simulink library "HexapodLib"  (R2014b)
settings: Solver=ode45  StartTime=0.0  StopTime=10.0  RelTol=1e-3
undefined symbols (not defined in the file): X, Y, Z
libraries: nesl_utility x95, sm_lib x85, HexapodLib x15, Contact_Forces_Lib x12
(part 1 of 3)
settings Model: Creator=Sebastian  LastModifiedBy=Sebastian

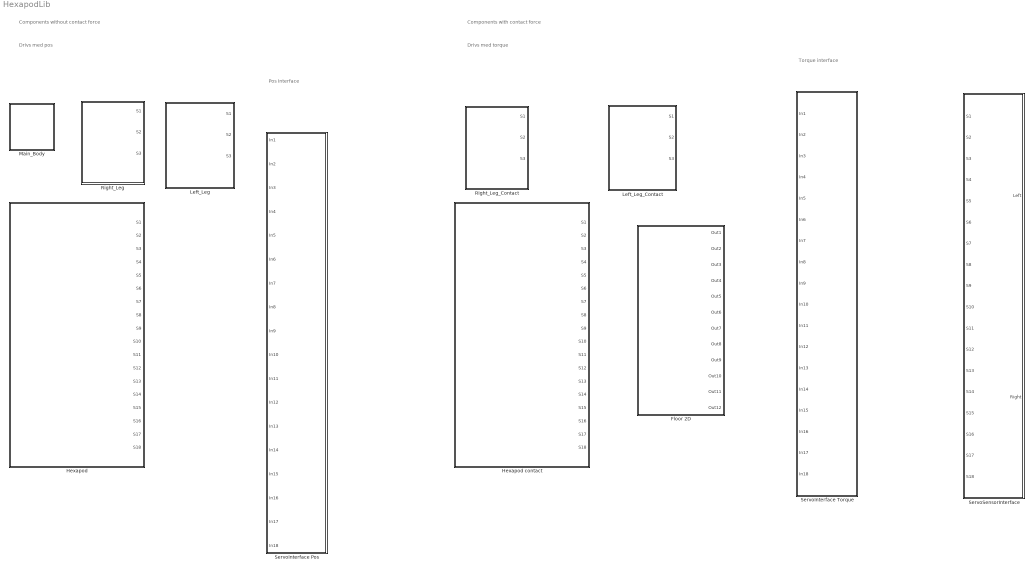
== system HexapodLib ==
  note: Pos Interface
  note: Torque interface
  note: Drivs med pos
  note: Components with contact force
  note: Components without contact force
  note: Drivs med torque
  Floor 2D : Subsystem  mask{my_k=0.5, my_s=0.7, v_th=0.0001}
      mask prompts: my_k "Coefficient of Kinetic Friction"; my_s "Coefficient of Static Friction"; v_th "Velocity Threshold (m/s)"
  Hexapod : Subsystem
  Hexapod contact : Subsystem
  Left_Leg : Subsystem
  Left_Leg_Contact : Subsystem
  Main_Body : Subsystem
  Right_Leg : Subsystem
  Right_Leg_Contact : Subsystem
  ServoInterface Pos : Subsystem  mask{Filter_time=0.001}
      mask prompts: Filter_time "Filter time"
  ServoInterface Torque : Subsystem
  ServoSensorInterface : Subsystem

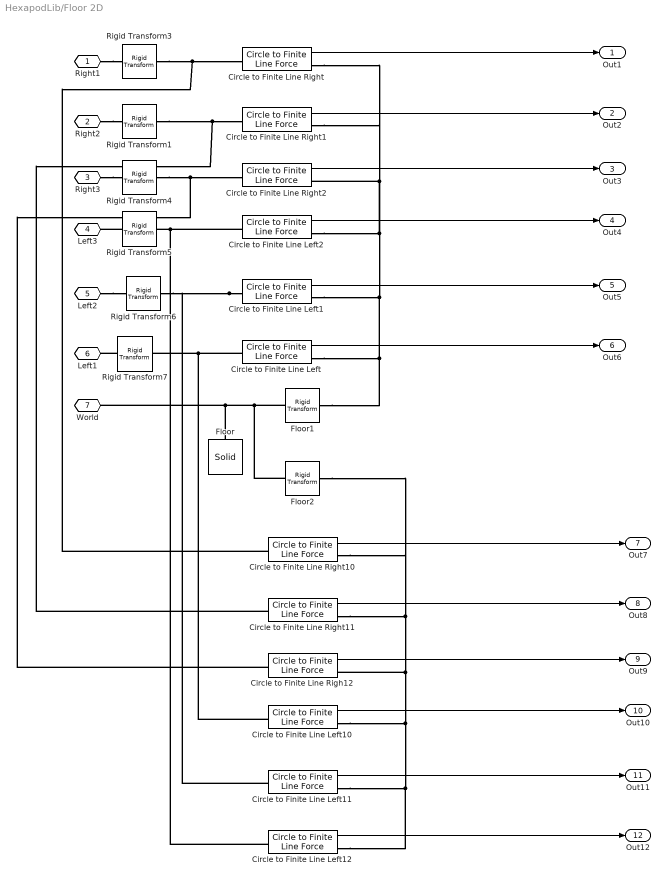
== system HexapodLib/Floor 2D ==
  Circle to Finite Line Left{,1..2,10..12} (6 alike) : Contact_Forces_Lib/2D/Circle to Finite Line Force  circle_rad=0.0048  line_depth=0.05/2  line_length=5  force_law=Linear  k_contact=1e6  b_contact=1e2  pen_full_damp_F=1e-2  pen_exponent=1  custom_param_1=1  custom_param_2=1  friction_law=Stick-Slip Continuous  mu_kinetic=my_k  mu_static=my_s  v_thr=v_th
  Circle to Finite Line Righ12 : Contact_Forces_Lib/2D/Circle to Finite Line Force  circle_rad=0.0048  line_depth=0.05/2  line_length=5  force_law=Linear  k_contact=1e6  b_contact=1e2  pen_full_damp_F=1e-2  pen_exponent=1  custom_param_1=1  custom_param_2=1  friction_law=Stick-Slip Continuous  mu_kinetic=my_k  mu_static=my_s  v_thr=v_th
  Circle to Finite Line Right{,1..2,10..11} (5 alike) : Contact_Forces_Lib/2D/Circle to Finite Line Force  circle_rad=0.0048  line_depth=0.05/2  line_length=5  force_law=Linear  k_contact=1e6  b_contact=1e2  pen_full_damp_F=1e-2  pen_exponent=1  custom_param_1=1  custom_param_2=1  friction_law=Stick-Slip Continuous  mu_kinetic=my_k  mu_static=my_s  v_thr=v_th
  Floor : sm_lib/Body Elements/Solid  InertiaType=CalculateFromGeometry  Mass=1  MassUnits=kg  CenterOfMass=[0 0 0]  CenterOfMassUnits=m  MomentsOfInertia=[1 1 1]  MomentsOfInertiaUnits=kg*m^2  ProductsOfInertia=[0 0 0]  ProductsOfInertiaUnits=kg*m^2  DensityBased=on  Density=1000  DensityUnits=kg/(m^3)  GraphicType=FromGeometry  MarkerShape=Sphere  MarkerSize=10  MarkerSizeUnits=m  GraphicVisPropType=SimpleVisualProperties  GraphicDiffuseColor=[0.4 0.4 0.0]  GraphicSpecularColor=[0.5 0.5 0.5 1.0]  GraphicAmbientColor=[0.15 0.15 0.15 1.0]  GraphicEmissiveColor=[0.0 0.0 0.0 1.0]  GraphicShininess=75  GraphicOpacity=1.0  GeometryShape=Brick  RectangleSize=[1 1]  RectangleSizeUnits=m  BrickDimensions=[3 3 0.05]  BrickDimensionUnits=m  CylinderRadius=1  CylinderRadiusUnits=m  CylinderLength=1  CylinderLengthUnits=m  SphereRadius=1  SphereRadiusUnits=m  EllipsoidRadii=[1 1 1]  EllipsoidRadiiUnits=m  ExtrusionCrossSection=[1 1; -1 1; -1 -1; 1 -1]  ExtrusionCrossSectionUnits=m  ExtrusionLength=1  ExtrusionLengthUnits=m  PolygonNumSides=3  PolygonOuterRadius=1  PolygonOuterRadiusUnits=m  ExtGeomFileType=STL  ExtGeomFileUnits=m  RevolutionCrossSection=[1 1; 1 -1; 2 -1; 2 1]  RevolutionCrossSectionUnits=m  RevolutionExtent=Full  RevolutionAngle=180  RevolutionAngleUnits=deg  BlockFunction=simmechanics.library.body_elements.solid
  Floor1 : sm_lib/Frames and Transforms/Rigid Transform  TranslationMethod=None  TranslationLengthUnit=m  TranslationStandardAxis=+Z  TranslationStandardOffset=0  TranslationCartesianOffset=[0 0 0]  TranslationROffset=0  TranslationROffsetUnits=m  TranslationZOffset=0  TranslationZOffsetUnits=m  TranslationThetaOffset=0  TranslationThetaOffsetUnits=deg  RotationMethod=AlignedAxes  RotationAngleUnits=deg  RotationStandardAxis=+Z  RotationAngle=0  RotationArbitraryAxis=[0 0 1]  FollAlignAxisA=+X  BaseAlignAxisA=+Z  FollAlignAxisB=+Y  BaseAlignAxisB=+X  RotationMatrix=[1 0 0; 0 1 0; 0 0 1]  BlockFunction=simmechanics.library.frames_transforms.rigid_transform
  Floor2 : sm_lib/Frames and Transforms/Rigid Transform  TranslationMethod=None  TranslationLengthUnit=m  TranslationStandardAxis=+Z  TranslationStandardOffset=0  TranslationCartesianOffset=[0 0 0]  TranslationROffset=0  TranslationROffsetUnits=m  TranslationZOffset=0  TranslationZOffsetUnits=m  TranslationThetaOffset=0  TranslationThetaOffsetUnits=deg  RotationMethod=AlignedAxes  RotationAngleUnits=deg  RotationStandardAxis=+Z  RotationAngle=0  RotationArbitraryAxis=[0 0 1]  FollAlignAxisA=+X  BaseAlignAxisA=+Z  FollAlignAxisB=+Y  BaseAlignAxisB=+Y  RotationMatrix=[1 0 0; 0 1 0; 0 0 1]  BlockFunction=simmechanics.library.frames_transforms.rigid_transform
  Rigid Transform{1,3..7} (6 alike) : sm_lib/Frames and Transforms/Rigid Transform  TranslationMethod=None  TranslationLengthUnit=m  TranslationStandardAxis=+Z  TranslationStandardOffset=0  TranslationCartesianOffset=[0 0 0]  TranslationROffset=0  TranslationROffsetUnits=m  TranslationZOffset=0  TranslationZOffsetUnits=m  TranslationThetaOffset=0  TranslationThetaOffsetUnits=deg  RotationMethod=StandardAxis  RotationAngleUnits=deg  RotationStandardAxis=+X  RotationAngle=90  RotationArbitraryAxis=[0 0 1]  FollAlignAxisA=+X  BaseAlignAxisA=+Z  FollAlignAxisB=+Y  BaseAlignAxisB=+X  RotationMatrix=[1 0 0; 0 1 0; 0 0 1]  BlockFunction=simmechanics.library.frames_transforms.rigid_transform
  Right1 : PMIOPort  Port=1  Side=Left
  Right2 : PMIOPort  Port=2  Side=Left
  Right3 : PMIOPort  Port=3  Side=Left
  Left3 : PMIOPort  Port=4  Side=Left
  Left2 : PMIOPort  Port=5  Side=Left
  Left1 : PMIOPort  Port=6  Side=Left
  World : PMIOPort  Port=7  Side=Left
  Out1 : Outport
  Out2 : Outport  Port=2
  Out3 : Outport  Port=3
  Out4 : Outport  Port=4
  Out5 : Outport  Port=5
  Out6 : Outport  Port=6
  Out7 : Outport  Port=7
  Out8 : Outport  Port=8
  Out9 : Outport  Port=9
  Out10 : Outport  Port=10
  Out11 : Outport  Port=11
  Out12 : Outport  Port=12
  wires:
  Circle to Finite Line Left12/1 -> Out12/1
  Circle to Finite Line Left11/1 -> Out11/1
  Circle to Finite Line Left10/1 -> Out10/1
  Circle to Finite Line Righ12/1 -> Out9/1
  Circle to Finite Line Right11/1 -> Out8/1
  Circle to Finite Line Right10/1 -> Out7/1
  Circle to Finite Line Left/1 -> Out6/1
  Circle to Finite Line Left1/1 -> Out5/1
  Circle to Finite Line Left2/1 -> Out4/1
  Circle to Finite Line Right2/1 -> Out3/1
  Circle to Finite Line Right1/1 -> Out2/1
  Circle to Finite Line Right/1 -> Out1/1
  connections:
  Circle to Finite Line Right10/RConn1 -- Floor2/RConn1 -- Circle to Finite Line Left11/RConn1 -- Circle to Finite Line Left12/RConn1 -- Circle to Finite Line Left10/RConn1 -- Circle to Finite Line Righ12/RConn1 -- Circle to Finite Line Right11/RConn1
  Floor1/LConn1 -- Floor/RConn1 -- World/RConn1 -- Floor2/LConn1
  Circle to Finite Line Left/LConn1 -- Rigid Transform7/RConn1 -- Circle to Finite Line Left10/LConn1
  Circle to Finite Line Left2/LConn1 -- Circle to Finite Line Left12/LConn1 -- Rigid Transform5/RConn1
  Circle to Finite Line Left1/LConn1 -- Rigid Transform6/RConn1 -- Circle to Finite Line Left11/LConn1
  Right1/RConn1 -- Rigid Transform3/LConn1
  Right2/RConn1 -- Rigid Transform1/LConn1
  Circle to Finite Line Righ12/LConn1 -- Rigid Transform4/RConn1 -- Circle to Finite Line Right2/LConn1
  Floor1/RConn1 -- Circle to Finite Line Left2/RConn1 -- Circle to Finite Line Right1/RConn1 -- Circle to Finite Line Right/RConn1 -- Circle to Finite Line Right2/RConn1 -- Circle to Finite Line Left1/RConn1 -- Circle to Finite Line Left/RConn1
  Rigid Transform3/RConn1 -- Circle to Finite Line Right10/LConn1 -- Circle to Finite Line Right/LConn1
  Rigid Transform1/RConn1 -- Circle to Finite Line Right11/LConn1 -- Circle to Finite Line Right1/LConn1
  Right3/RConn1 -- Rigid Transform4/LConn1
  Rigid Transform5/LConn1 -- Left3/RConn1
  Left2/RConn1 -- Rigid Transform6/LConn1
  Rigid Transform7/LConn1 -- Left1/RConn1

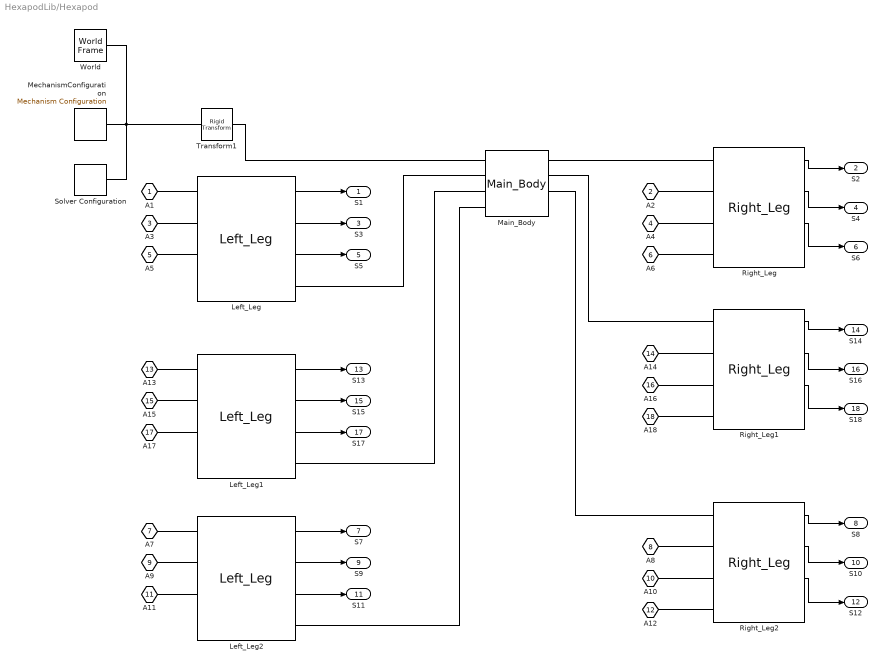
== system HexapodLib/Hexapod ==
  Left_Leg : HexapodLib/Left_Leg  SystemSampleTime=-1
  Left_Leg1 : HexapodLib/Left_Leg  SystemSampleTime=-1
  Left_Leg2 : HexapodLib/Left_Leg  SystemSampleTime=-1
  Main_Body : HexapodLib/Main_Body  SystemSampleTime=-1
  MechanismConfiguration : sm_lib/Utilities/Mechanism Configuration  UniformGravity=Constant  GravityVector=[0 0 -9.81]  GravityUnits=m/s^2  LinearizationDelta=0.001  BlockFunction=simmechanics.library.utilities.mechanism_configuration
  Right_Leg : HexapodLib/Right_Leg  SystemSampleTime=-1
  Right_Leg1 : HexapodLib/Right_Leg  SystemSampleTime=-1
  Right_Leg2 : HexapodLib/Right_Leg  SystemSampleTime=-1
  Solver Configuration : nesl_utility/Solver Configuration  PhysicalDomain=network_engine_domain  SubClassName=solver  LeftPortType=input  RightPortType=generic  Accelerate=off  Tones=[]  Harmonics=[]  SimulateNoise=off  Profile=off  UseLocalSampling=off  EnableSwitchedLinearOptims=on  FrequencyDomain=off  UseCCode=off  RelTol=0.001  AbsTol=1e-06  MinStep=1e-09  ToWorkspace=off  DoDC=off  ResidualTolerance=1e-09  UseLocalSolver=off  LocalSolverChoice=NE_BACKWARD_EULER_ADVANCER  LocalSolverSampleTime=0.001  DoFixedCost=off  MaxNonlinIter=3  MaxModeIter=2  LinearAlgebra=Sparse  DelaysMemoryBudget=1024  AutomaticFiltering=on  FilteringTimeConstant=0.001
  Transform1 : sm_lib/Frames and Transforms/Rigid Transform  TranslationMethod=Cartesian  TranslationLengthUnit=cm  TranslationStandardAxis=+Z  TranslationStandardOffset=0  TranslationCartesianOffset=[0 0 17]  TranslationROffset=0  TranslationROffsetUnits=m  TranslationZOffset=0  TranslationZOffsetUnits=m  TranslationThetaOffset=0  TranslationThetaOffsetUnits=deg  RotationMethod=StandardAxis  RotationAngleUnits=deg  RotationStandardAxis=+Z  RotationAngle=180  RotationArbitraryAxis=[0 0 0]  FollAlignAxisA=+X  BaseAlignAxisA=+Y  FollAlignAxisB=+Y  BaseAlignAxisB=+Z  RotationMatrix=[1 0 0; 0 1 0; 0 0 1]  BlockFunction=simmechanics.library.frames_transforms.rigid_transform
  World : sm_lib/Frames and Transforms/World Frame  BlockFunction=simmechanics.library.frames_transforms.world_frame
  A1 : PMIOPort  Port=1  Side=Left
  A2 : PMIOPort  Port=2  Side=Left
  A3 : PMIOPort  Port=3  Side=Left
  A4 : PMIOPort  Port=4  Side=Left
  A5 : PMIOPort  Port=5  Side=Left
  A6 : PMIOPort  Port=6  Side=Left
  A7 : PMIOPort  Port=7  Side=Left
  A8 : PMIOPort  Port=8  Side=Left
  A9 : PMIOPort  Port=9  Side=Left
  A10 : PMIOPort  Port=10  Side=Left
  A11 : PMIOPort  Port=11  Side=Left
  A12 : PMIOPort  Port=12  Side=Left
  A13 : PMIOPort  Port=13  Side=Left
  A14 : PMIOPort  Port=14  Side=Left
  A15 : PMIOPort  Port=15  Side=Left
  A16 : PMIOPort  Port=16  Side=Left
  A17 : PMIOPort  Port=17  Side=Left
  A18 : PMIOPort  Port=18  Side=Left
  S1 : Outport
  S2 : Outport  Port=2
  S3 : Outport  Port=3
  S4 : Outport  Port=4
  S5 : Outport  Port=5
  S6 : Outport  Port=6
  S7 : Outport  Port=7
  S8 : Outport  Port=8
  S9 : Outport  Port=9
  S10 : Outport  Port=10
  S11 : Outport  Port=11
  S12 : Outport  Port=12
  S13 : Outport  Port=13
  S14 : Outport  Port=14
  S15 : Outport  Port=15
  S16 : Outport  Port=16
  S17 : Outport  Port=17
  S18 : Outport  Port=18
  wires:
  Right_Leg/3 -> S6/1
  Right_Leg/2 -> S4/1
  Right_Leg/1 -> S2/1
  Left_Leg/1 -> S1/1
  Left_Leg/2 -> S3/1
  Left_Leg/3 -> S5/1
  Left_Leg1/1 -> S13/1
  Left_Leg1/2 -> S15/1
  Left_Leg1/3 -> S17/1
  Left_Leg2/1 -> S7/1
  Left_Leg2/2 -> S9/1
  Left_Leg2/3 -> S11/1
  Right_Leg2/1 -> S8/1
  Right_Leg2/2 -> S10/1
  Right_Leg2/3 -> S12/1
  Right_Leg1/1 -> S14/1
  Right_Leg1/2 -> S16/1
  Right_Leg1/3 -> S18/1
  connections:
  Main_Body/LConn4 -- Left_Leg2/RConn1
  Main_Body/LConn1 -- Transform1/RConn1
  Main_Body/LConn2 -- Left_Leg/RConn1
  A4/RConn1 -- Right_Leg/LConn3
  Main_Body/RConn2 -- Right_Leg1/LConn1
  A2/RConn1 -- Right_Leg/LConn2
  A6/RConn1 -- Right_Leg/LConn4
  Main_Body/LConn3 -- Left_Leg1/RConn1
  Solver Configuration/RConn1 -- Transform1/LConn1 -- MechanismConfiguration/RConn1 -- World/RConn1
  Main_Body/RConn1 -- Right_Leg/LConn1
  Main_Body/RConn3 -- Right_Leg2/LConn1
  A8/RConn1 -- Right_Leg2/LConn2
  A10/RConn1 -- Right_Leg2/LConn3
  A12/RConn1 -- Right_Leg2/LConn4
  A14/RConn1 -- Right_Leg1/LConn2
  A16/RConn1 -- Right_Leg1/LConn3
  A18/RConn1 -- Right_Leg1/LConn4
  A1/RConn1 -- Left_Leg/LConn1
  A3/RConn1 -- Left_Leg/LConn2
  A5/RConn1 -- Left_Leg/LConn3
  A13/RConn1 -- Left_Leg1/LConn1
  A15/RConn1 -- Left_Leg1/LConn2
  A17/RConn1 -- Left_Leg1/LConn3
  A7/RConn1 -- Left_Leg2/LConn1
  A9/RConn1 -- Left_Leg2/LConn2
  A11/RConn1 -- Left_Leg2/LConn3

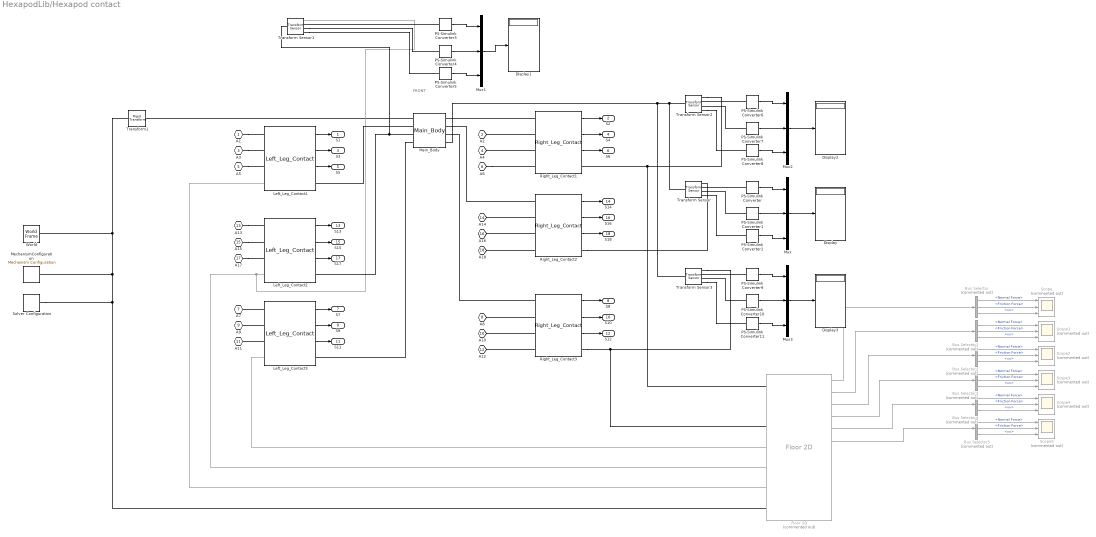
== system HexapodLib/Hexapod contact ==
  note: FRONT
  Bus Selector{,1..5} (6 alike) : BusSelector  Commented=on  OutputSignals=Normal Force,Friction Force,Frame Sep.vx
  Display{,1..3} (4 alike) : Display
  Floor 2D : HexapodLib/Floor 2D  Commented=on  my_k=0.5  my_s=0.7  v_th=0.01
  Left_Leg_Contact1 : HexapodLib/Left_Leg_Contact  SystemSampleTime=-1
  Left_Leg_Contact2 : HexapodLib/Left_Leg_Contact  SystemSampleTime=-1
  Left_Leg_Contact3 : HexapodLib/Left_Leg_Contact  SystemSampleTime=-1
  Main_Body : HexapodLib/Main_Body  SystemSampleTime=-1
  MechanismConfiguration : sm_lib/Utilities/Mechanism Configuration  UniformGravity=Constant  GravityVector=[0 0 -9.81]  GravityUnits=m/s^2  LinearizationDelta=0.001  BlockFunction=simmechanics.library.utilities.mechanism_configuration
  Mux{,1..3} (4 alike) : Mux  Inputs=3
  PS-Simulink Converter{,1..11} (12 alike) : nesl_utility/PS-Simulink Converter  PhysicalDomain=network_engine_domain  SubClassName=ps_output  LeftPortType=input  RightPortType=output  PseudoPeriodic=off  Frequencies=[]  Unit=mm  AffineConversion=off
  Right_Leg_Contact1 : HexapodLib/Right_Leg_Contact  SystemSampleTime=-1
  Right_Leg_Contact2 : HexapodLib/Right_Leg_Contact  SystemSampleTime=-1
  Right_Leg_Contact3 : HexapodLib/Right_Leg_Contact  SystemSampleTime=-1
  Scope{,1..5} (6 alike) : Scope  Commented=on  NumInputPorts=3
      Scope settings: YMin=0.5~2e-05~-1.1e-06  YMax=2~0.00011~-4e-07
      Scope1 settings: YMin=-5~-5~-5  YMax=5~5~5
      Scope2 settings: YMin=-5~-5~-5  YMax=5~5~5
      Scope3 settings: YMin=-5~-5~-5  YMax=5~5~5  SaveName=ScopeData2
      Scope4 settings: YMin=-5~-5~-5  YMax=5~5~5  SaveName=ScopeData3
      Scope5 settings: YMin=-5~-5~-5  YMax=5~5~5  SaveName=ScopeData4
  Solver Configuration : nesl_utility/Solver Configuration  PhysicalDomain=network_engine_domain  SubClassName=solver  LeftPortType=input  RightPortType=generic  Accelerate=off  Tones=[]  Harmonics=[]  SimulateNoise=off  Profile=off  UseLocalSampling=off  EnableSwitchedLinearOptims=on  FrequencyDomain=off  UseCCode=off  RelTol=0.001  AbsTol=1e-06  MinStep=1e-09  ToWorkspace=off  DoDC=off  ResidualTolerance=1e-09  UseLocalSolver=off  LocalSolverChoice=NE_BACKWARD_EULER_ADVANCER  LocalSolverSampleTime=0.001  DoFixedCost=off  MaxNonlinIter=3  MaxModeIter=2  LinearAlgebra=Sparse  DelaysMemoryBudget=1024  AutomaticFiltering=on  FilteringTimeConstant=0.001
  Transform Sensor{,1..3} (4 alike) : sm_lib/Frames and Transforms/Transform Sensor  MeasurementFrame=Base  SenseAngle=off  SenseAxis=off  SenseAngle1=off  SenseAngle2=off  SenseAngle3=off  SenseQ=off  SenseR=off  SenseOmegaX=off  SenseOmegaY=off  SenseOmegaZ=off  SenseOmega1=off  SenseOmega2=off  SenseOmega3=off  SenseQDot=off  SenseRDot=off  SenseAlphaX=off  SenseAlphaY=off  SenseAlphaZ=off  SenseAlpha1=off  SenseAlpha2=off  SenseAlpha3=off  SenseQDDot=off  SenseRDDot=off  SenseX=on  SenseY=on  SenseZ=on  SenseRad=off  SenseAzim=off  SenseDist=off  SenseInc=off  SenseXDot=off  SenseYDot=off  SenseZDot=off  SenseRadDot=off  SenseAzimDot=off  SenseDistDot=off  SenseIncDot=off  SenseXDDot=off  SenseYDDot=off  SenseZDDot=off  SenseRadDDot=off  SenseAzimDDot=off  SenseDistDDot=off  SenseIncDDot=off  BlockFunction=simmechanics.library.frames_transforms.transform_sensor
  Transform1 : sm_lib/Frames and Transforms/Rigid Transform  TranslationMethod=Cartesian  TranslationLengthUnit=cm  TranslationStandardAxis=+Z  TranslationStandardOffset=0  TranslationCartesianOffset=[0 0 17]  TranslationROffset=0  TranslationROffsetUnits=m  TranslationZOffset=0  TranslationZOffsetUnits=m  TranslationThetaOffset=0  TranslationThetaOffsetUnits=deg  RotationMethod=StandardAxis  RotationAngleUnits=deg  RotationStandardAxis=+Z  RotationAngle=180  RotationArbitraryAxis=[0 0 0]  FollAlignAxisA=+X  BaseAlignAxisA=+Y  FollAlignAxisB=+Y  BaseAlignAxisB=+Z  RotationMatrix=[1 0 0; 0 1 0; 0 0 1]  BlockFunction=simmechanics.library.frames_transforms.rigid_transform
  World : sm_lib/Frames and Transforms/World Frame  BlockFunction=simmechanics.library.frames_transforms.world_frame
  A1 : PMIOPort  Port=1  Side=Left
  A2 : PMIOPort  Port=2  Side=Left
  A3 : PMIOPort  Port=3  Side=Left
  A4 : PMIOPort  Port=4  Side=Left
  A5 : PMIOPort  Port=5  Side=Left
  A6 : PMIOPort  Port=6  Side=Left
  A7 : PMIOPort  Port=7  Side=Left
  A8 : PMIOPort  Port=8  Side=Left
  A9 : PMIOPort  Port=9  Side=Left
  A10 : PMIOPort  Port=10  Side=Left
  A11 : PMIOPort  Port=11  Side=Left
  A12 : PMIOPort  Port=12  Side=Left
  A13 : PMIOPort  Port=13  Side=Left
  A14 : PMIOPort  Port=14  Side=Left
  A15 : PMIOPort  Port=15  Side=Left
  A16 : PMIOPort  Port=16  Side=Left
  A17 : PMIOPort  Port=17  Side=Left
  A18 : PMIOPort  Port=18  Side=Left
  S1 : Outport
  S2 : Outport  Port=2
  S3 : Outport  Port=3
  S4 : Outport  Port=4
  S5 : Outport  Port=5
  S6 : Outport  Port=6
  S7 : Outport  Port=7
  S8 : Outport  Port=8
  S9 : Outport  Port=9
  S10 : Outport  Port=10
  S11 : Outport  Port=11
  S12 : Outport  Port=12
  S13 : Outport  Port=13
  S14 : Outport  Port=14
  S15 : Outport  Port=15
  S16 : Outport  Port=16
  S17 : Outport  Port=17
  S18 : Outport  Port=18
  wires:
  PS-Simulink Converter9/1 -> Mux3/1
  PS-Simulink Converter10/1 -> Mux3/2
  PS-Simulink Converter11/1 -> Mux3/3
  Mux3/1 -> Display3/1
  PS-Simulink Converter6/1 -> Mux2/1
  PS-Simulink Converter7/1 -> Mux2/2
  PS-Simulink Converter8/1 -> Mux2/3
  Mux2/1 -> Display2/1
  Left_Leg_Contact3/3 -> S11/1
  Left_Leg_Contact3/2 -> S9/1
  Left_Leg_Contact3/1 -> S7/1
  Left_Leg_Contact2/3 -> S17/1
  Left_Leg_Contact2/2 -> S15/1
  Left_Leg_Contact2/1 -> S13/1
  Left_Leg_Contact1/3 -> S5/1
  Floor 2D/6 -> Bus Selector5/1
  Floor 2D/5 -> Bus Selector4/1
  Floor 2D/4 -> Bus Selector3/1
  Floor 2D/3 -> Bus Selector2/1
  Floor 2D/2 -> Bus Selector1/1
  Floor 2D/1 -> Bus Selector/1
  Left_Leg_Contact1/1 -> S1/1
  Left_Leg_Contact1/2 -> S3/1
  Right_Leg_Contact1/1 -> S2/1
  Right_Leg_Contact1/2 -> S4/1
  Right_Leg_Contact1/3 -> S6/1
  Bus Selector/1 -> Scope/1  "<Normal Force>"
  Bus Selector/2 -> Scope/2  "<Friction Force>"
  Bus Selector/3 -> Scope/3  "<vx>"
  Bus Selector1/1 -> Scope1/1  "<Normal Force>"
  Bus Selector1/2 -> Scope1/2  "<Friction Force>"
  Bus Selector1/3 -> Scope1/3  "<vx>"
  Bus Selector2/1 -> Scope2/1  "<Normal Force>"
  Bus Selector2/2 -> Scope2/2  "<Friction Force>"
  Bus Selector2/3 -> Scope2/3  "<vx>"
  Bus Selector3/1 -> Scope3/1  "<Normal Force>"
  Bus Selector3/2 -> Scope3/2  "<Friction Force>"
  Bus Selector3/3 -> Scope3/3  "<vx>"
  Bus Selector4/1 -> Scope4/1  "<Normal Force>"
  Bus Selector4/2 -> Scope4/2  "<Friction Force>"
  Bus Selector4/3 -> Scope4/3  "<vx>"
  Bus Selector5/1 -> Scope5/1  "<Normal Force>"
  Bus Selector5/2 -> Scope5/2  "<Friction Force>"
  Bus Selector5/3 -> Scope5/3  "<vx>"
  Right_Leg_Contact3/1 -> S8/1
  Right_Leg_Contact3/2 -> S10/1
  Right_Leg_Contact3/3 -> S12/1
  Right_Leg_Contact2/1 -> S14/1
  Right_Leg_Contact2/2 -> S16/1
  Right_Leg_Contact2/3 -> S18/1
  PS-Simulink Converter/1 -> Mux/1
  PS-Simulink Converter1/1 -> Mux/2
  PS-Simulink Converter2/1 -> Mux/3
  Mux/1 -> Display/1
  PS-Simulink Converter3/1 -> Mux1/1
  PS-Simulink Converter4/1 -> Mux1/2
  PS-Simulink Converter5/1 -> Mux1/3
  Mux1/1 -> Display1/1
  connections:
  Right_Leg_Contact3/LConn1 -- Main_Body/RConn3
  Main_Body/RConn4 -- Transform Sensor3/LConn1 -- Transform Sensor/LConn1 -- Transform Sensor2/LConn1
  PS-Simulink Converter10/LConn1 -- Transform Sensor3/RConn3
  PS-Simulink Converter9/LConn1 -- Transform Sensor3/RConn2
  Transform Sensor3/RConn4 -- PS-Simulink Converter11/LConn1
  PS-Simulink Converter7/LConn1 -- Transform Sensor2/RConn3
  Transform Sensor2/RConn4 -- PS-Simulink Converter8/LConn1
  PS-Simulink Converter6/LConn1 -- Transform Sensor2/RConn2
  Main_Body/LConn1 -- Transform1/RConn1
  Left_Leg_Contact3/LConn3 -- A11/RConn1
  Left_Leg_Contact3/LConn2 -- A9/RConn1
  Left_Leg_Contact3/LConn1 -- A7/RConn1
  A17/RConn1 -- Left_Leg_Contact2/LConn3
  A15/RConn1 -- Left_Leg_Contact2/LConn2
  A13/RConn1 -- Left_Leg_Contact2/LConn1
  A5/RConn1 -- Left_Leg_Contact1/LConn3
  A3/RConn1 -- Left_Leg_Contact1/LConn2
  A1/RConn1 -- Left_Leg_Contact1/LConn1
  Transform Sensor3/RConn1 -- Floor 2D/LConn3 -- Right_Leg_Contact3/RConn1
  Transform Sensor2/RConn1 -- Right_Leg_Contact1/RConn1 -- Floor 2D/LConn1
  Right_Leg_Contact2/LConn3 -- A16/RConn1
  Right_Leg_Contact2/LConn2 -- A14/RConn1
  Right_Leg_Contact3/LConn3 -- A10/RConn1
  Right_Leg_Contact3/LConn2 -- A8/RConn1
  Right_Leg_Contact1/LConn1 -- Main_Body/RConn1
  Transform1/LConn1 -- World/RConn1 -- MechanismConfiguration/RConn1 -- Solver Configuration/RConn1 -- Floor 2D/LConn7
  Right_Leg_Contact1/LConn2 -- A2/RConn1
  Right_Leg_Contact2/LConn1 -- Main_Body/RConn2
  Right_Leg_Contact1/LConn3 -- A4/RConn1
  Right_Leg_Contact3/LConn4 -- A12/RConn1
  Right_Leg_Contact2/LConn4 -- A18/RConn1
  A6/RConn1 -- Right_Leg_Contact1/LConn4
  Floor 2D/LConn6 -- Left_Leg_Contact1/LConn4
  Floor 2D/LConn5 -- Transform Sensor1/RConn1 -- Left_Leg_Contact2/LConn4
  Floor 2D/LConn4 -- Left_Leg_Contact3/LConn4
  Main_Body/LConn2 -- Left_Leg_Contact1/RConn1
  Main_Body/LConn3 -- Transform Sensor1/LConn1 -- Left_Leg_Contact2/RConn1
  Main_Body/LConn4 -- Left_Leg_Contact3/RConn1
  Right_Leg_Contact2/RConn1 -- Transform Sensor/RConn1
  PS-Simulink Converter/LConn1 -- Transform Sensor/RConn2
  PS-Simulink Converter1/LConn1 -- Transform Sensor/RConn3
  Transform Sensor/RConn4 -- PS-Simulink Converter2/LConn1
  Transform Sensor1/RConn4 -- PS-Simulink Converter5/LConn1
  PS-Simulink Converter3/LConn1 -- Transform Sensor1/RConn2
  Transform Sensor1/RConn3 -- PS-Simulink Converter4/LConn1

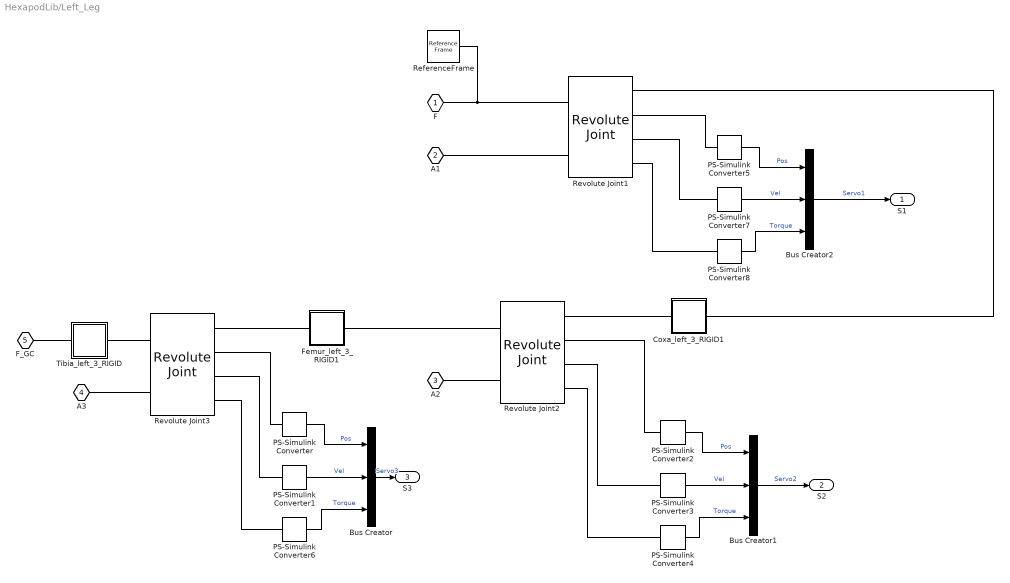
== system HexapodLib/Left_Leg ==
  Bus Creator : BusCreator  Inputs=3  OutDataTypeStr=Bus: Mes_servo
      settings: InheritFromInputs=off
  Bus Creator1 : BusCreator  Inputs=3  OutDataTypeStr=Bus: Mes_servo
      settings: InheritFromInputs=off
  Bus Creator2 : BusCreator  Inputs=3  OutDataTypeStr=Bus: Mes_servo
      settings: InheritFromInputs=off
  Coxa_left_3_RIGID1 : Subsystem
  Femur_left_3_RIGID1 : Subsystem
  PS-Simulink Converter : nesl_utility/PS-Simulink Converter  PhysicalDomain=network_engine_domain  SubClassName=ps_output  LeftPortType=input  RightPortType=output  PseudoPeriodic=off  Frequencies=[]  Unit=rad  AffineConversion=off
  PS-Simulink Converter1 : nesl_utility/PS-Simulink Converter  PhysicalDomain=network_engine_domain  SubClassName=ps_output  LeftPortType=input  RightPortType=output  PseudoPeriodic=off  Frequencies=[]  Unit=rad/s  AffineConversion=off
  PS-Simulink Converter2 : nesl_utility/PS-Simulink Converter  PhysicalDomain=network_engine_domain  SubClassName=ps_output  LeftPortType=input  RightPortType=output  PseudoPeriodic=off  Frequencies=[]  Unit=rad  AffineConversion=off
  PS-Simulink Converter3 : nesl_utility/PS-Simulink Converter  PhysicalDomain=network_engine_domain  SubClassName=ps_output  LeftPortType=input  RightPortType=output  PseudoPeriodic=off  Frequencies=[]  Unit=rad/s  AffineConversion=off
  PS-Simulink Converter4 : nesl_utility/PS-Simulink Converter  PhysicalDomain=network_engine_domain  SubClassName=ps_output  LeftPortType=input  RightPortType=output  PseudoPeriodic=off  Frequencies=[]  Unit=N*m  AffineConversion=off
  PS-Simulink Converter5 : nesl_utility/PS-Simulink Converter  PhysicalDomain=network_engine_domain  SubClassName=ps_output  LeftPortType=input  RightPortType=output  PseudoPeriodic=off  Frequencies=[]  Unit=rad  AffineConversion=off
  PS-Simulink Converter6 : nesl_utility/PS-Simulink Converter  PhysicalDomain=network_engine_domain  SubClassName=ps_output  LeftPortType=input  RightPortType=output  PseudoPeriodic=off  Frequencies=[]  Unit=N*m  AffineConversion=off
  PS-Simulink Converter7 : nesl_utility/PS-Simulink Converter  PhysicalDomain=network_engine_domain  SubClassName=ps_output  LeftPortType=input  RightPortType=output  PseudoPeriodic=off  Frequencies=[]  Unit=rad/s  AffineConversion=off
  PS-Simulink Converter8 : nesl_utility/PS-Simulink Converter  PhysicalDomain=network_engine_domain  SubClassName=ps_output  LeftPortType=input  RightPortType=output  PseudoPeriodic=off  Frequencies=[]  Unit=N*m  AffineConversion=off
  ReferenceFrame : sm_lib/Frames and Transforms/Reference Frame  BlockFunction=simmechanics.library.frames_transforms.reference_frame
  Revolute Joint1 : sm_lib/Joints/Revolute Joint  SenseConstraintForce=off  SenseConstraintForceX=off  SenseConstraintForceY=off  SenseConstraintForceZ=off  SenseConstraintTorque=off  SenseConstraintTorqueX=off  SenseConstraintTorqueY=off  SenseConstraintTorqueZ=off  SenseTotalForce=off  SenseTotalForceX=off  SenseTotalForceY=off  SenseTotalForceZ=off  SenseTotalTorque=off  SenseTotalTorqueX=off  SenseTotalTorqueY=off  SenseTotalTorqueZ=off  CompositeWrenchDir=FollowerOnBase  CompositeWrenchFrame=BaseFrame  EquilibriumPosition=0  EquilibriumPositionUnits=deg  SpringStiffness=spring_stiff  SpringStiffnessUnits=N*m/deg  DampingCoefficient=damping_coeff  DampingCoefficientUnits=N*m/(deg/s)  TorqueActuationMode=ComputedTorque  MotionActuationMode=InputMotion  SensePosition=on  SenseVelocity=on  SenseAcceleration=off  SenseTorqueForce=on  PositionTargetValue=0  PositionTargetValueUnits=deg  PositionTargetSpecify=off  PositionTargetPriority=High  VelocityTargetValue=0  VelocityTargetValueUnits=deg/s  VelocityTargetSpecify=off  VelocityTargetPriority=High  BlockFunction=simmechanics.library.joints.revolute_joint
  Revolute Joint2 : sm_lib/Joints/Revolute Joint  SenseConstraintForce=off  SenseConstraintForceX=off  SenseConstraintForceY=off  SenseConstraintForceZ=off  SenseConstraintTorque=off  SenseConstraintTorqueX=off  SenseConstraintTorqueY=off  SenseConstraintTorqueZ=off  SenseTotalForce=off  SenseTotalForceX=off  SenseTotalForceY=off  SenseTotalForceZ=off  SenseTotalTorque=off  SenseTotalTorqueX=off  SenseTotalTorqueY=off  SenseTotalTorqueZ=off  CompositeWrenchDir=FollowerOnBase  CompositeWrenchFrame=BaseFrame  EquilibriumPosition=0  EquilibriumPositionUnits=deg  SpringStiffness=spring_stiff  SpringStiffnessUnits=N*m/deg  DampingCoefficient=damping_coeff  DampingCoefficientUnits=N*m/(deg/s)  TorqueActuationMode=ComputedTorque  MotionActuationMode=InputMotion  SensePosition=on  SenseVelocity=on  SenseAcceleration=off  SenseTorqueForce=on  PositionTargetValue=0  PositionTargetValueUnits=deg  PositionTargetSpecify=off  PositionTargetPriority=High  VelocityTargetValue=0  VelocityTargetValueUnits=deg/s  VelocityTargetSpecify=off  VelocityTargetPriority=High  BlockFunction=simmechanics.library.joints.revolute_joint
  Revolute Joint3 : sm_lib/Joints/Revolute Joint  SenseConstraintForce=off  SenseConstraintForceX=off  SenseConstraintForceY=off  SenseConstraintForceZ=off  SenseConstraintTorque=off  SenseConstraintTorqueX=off  SenseConstraintTorqueY=off  SenseConstraintTorqueZ=off  SenseTotalForce=off  SenseTotalForceX=off  SenseTotalForceY=off  SenseTotalForceZ=off  SenseTotalTorque=off  SenseTotalTorqueX=off  SenseTotalTorqueY=off  SenseTotalTorqueZ=off  CompositeWrenchDir=FollowerOnBase  CompositeWrenchFrame=BaseFrame  EquilibriumPosition=0  EquilibriumPositionUnits=deg  SpringStiffness=spring_stiff  SpringStiffnessUnits=N*m/deg  DampingCoefficient=damping_coeff  DampingCoefficientUnits=N*m/(deg/s)  TorqueActuationMode=ComputedTorque  MotionActuationMode=InputMotion  SensePosition=on  SenseVelocity=on  SenseAcceleration=off  SenseTorqueForce=on  PositionTargetValue=0  PositionTargetValueUnits=deg  PositionTargetSpecify=off  PositionTargetPriority=High  VelocityTargetValue=0  VelocityTargetValueUnits=deg/s  VelocityTargetSpecify=off  VelocityTargetPriority=High  BlockFunction=simmechanics.library.joints.revolute_joint
  Tibia_left_3_RIGID : Subsystem
  F : PMIOPort  Port=1  Side=Right
  A1 : PMIOPort  Port=2  Side=Left
  A2 : PMIOPort  Port=3  Side=Left
  A3 : PMIOPort  Port=4  Side=Left
  F_GC : PMIOPort  Port=5  Side=Left
  S1 : Outport
  S2 : Outport  Port=2
  S3 : Outport  Port=3
  wires:
  Bus Creator/1 -> S3/1  "Servo3"
  PS-Simulink Converter1/1 -> Bus Creator/2  "Vel"
  PS-Simulink Converter/1 -> Bus Creator/1  "Pos"
  PS-Simulink Converter6/1 -> Bus Creator/3  "Torque"
  Bus Creator1/1 -> S2/1  "Servo2"
  PS-Simulink Converter3/1 -> Bus Creator1/2  "Vel"
  PS-Simulink Converter2/1 -> Bus Creator1/1  "Pos"
  PS-Simulink Converter4/1 -> Bus Creator1/3  "Torque"
  Bus Creator2/1 -> S1/1  "Servo1"
  PS-Simulink Converter7/1 -> Bus Creator2/2  "Vel"
  PS-Simulink Converter5/1 -> Bus Creator2/1  "Pos"
  PS-Simulink Converter8/1 -> Bus Creator2/3  "Torque"
  connections:
  A1/RConn1 -- Revolute Joint1/LConn2
  Coxa_left_3_RIGID1/LConn1 -- Revolute Joint1/RConn1
  ReferenceFrame/RConn1 -- Revolute Joint1/LConn1 -- F/RConn1
  F_GC/RConn1 -- Tibia_left_3_RIGID/RConn1
  Revolute Joint2/RConn1 -- Coxa_left_3_RIGID1/RConn1
  Revolute Joint3/LConn1 -- Tibia_left_3_RIGID/LConn1
  Revolute Joint3/RConn1 -- Femur_left_3_RIGID1/RConn1
  A2/RConn1 -- Revolute Joint2/LConn2
  PS-Simulink Converter2/LConn1 -- Revolute Joint2/RConn2
  PS-Simulink Converter3/LConn1 -- Revolute Joint2/RConn3
  PS-Simulink Converter4/LConn1 -- Revolute Joint2/RConn4
  A3/RConn1 -- Revolute Joint3/LConn2
  PS-Simulink Converter/LConn1 -- Revolute Joint3/RConn2
  PS-Simulink Converter1/LConn1 -- Revolute Joint3/RConn3
  PS-Simulink Converter6/LConn1 -- Revolute Joint3/RConn4
  Revolute Joint2/LConn1 -- Femur_left_3_RIGID1/LConn1
  PS-Simulink Converter8/LConn1 -- Revolute Joint1/RConn4
  PS-Simulink Converter7/LConn1 -- Revolute Joint1/RConn3
  PS-Simulink Converter5/LConn1 -- Revolute Joint1/RConn2

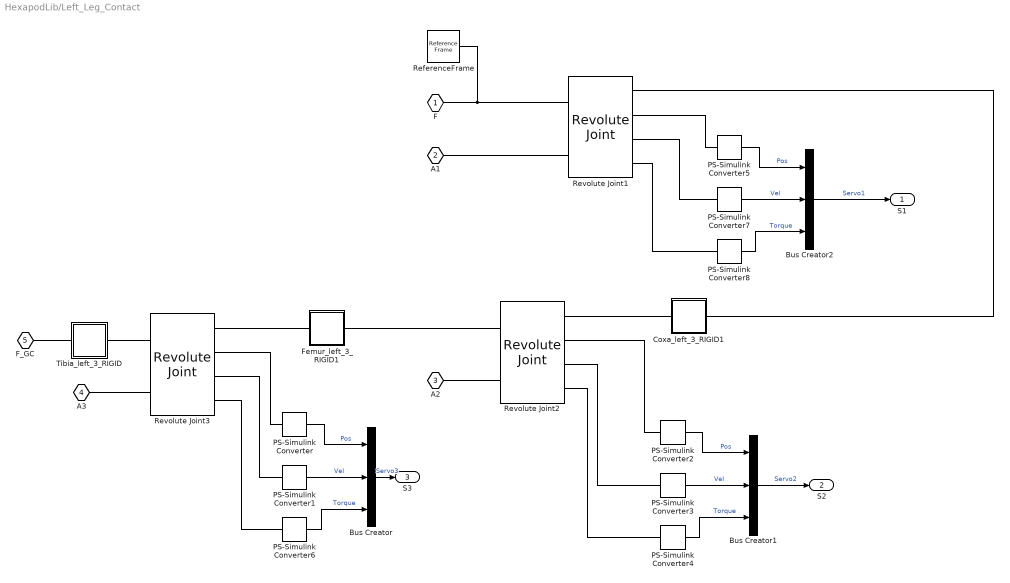
== system HexapodLib/Left_Leg_Contact ==
  Bus Creator : BusCreator  Inputs=3  OutDataTypeStr=Bus: Mes_servo
      settings: InheritFromInputs=off
  Bus Creator1 : BusCreator  Inputs=3  OutDataTypeStr=Bus: Mes_servo
      settings: InheritFromInputs=off
  Bus Creator2 : BusCreator  Inputs=3  OutDataTypeStr=Bus: Mes_servo
      settings: InheritFromInputs=off
  Coxa_left_3_RIGID1 : Subsystem
  Femur_left_3_RIGID1 : Subsystem
  PS-Simulink Converter : nesl_utility/PS-Simulink Converter  PhysicalDomain=network_engine_domain  SubClassName=ps_output  LeftPortType=input  RightPortType=output  PseudoPeriodic=off  Frequencies=[]  Unit=rad  AffineConversion=off
  PS-Simulink Converter1 : nesl_utility/PS-Simulink Converter  PhysicalDomain=network_engine_domain  SubClassName=ps_output  LeftPortType=input  RightPortType=output  PseudoPeriodic=off  Frequencies=[]  Unit=rad/s  AffineConversion=off
  PS-Simulink Converter2 : nesl_utility/PS-Simulink Converter  PhysicalDomain=network_engine_domain  SubClassName=ps_output  LeftPortType=input  RightPortType=output  PseudoPeriodic=off  Frequencies=[]  Unit=rad  AffineConversion=off
  PS-Simulink Converter3 : nesl_utility/PS-Simulink Converter  PhysicalDomain=network_engine_domain  SubClassName=ps_output  LeftPortType=input  RightPortType=output  PseudoPeriodic=off  Frequencies=[]  Unit=rad/s  AffineConversion=off
  PS-Simulink Converter4 : nesl_utility/PS-Simulink Converter  PhysicalDomain=network_engine_domain  SubClassName=ps_output  LeftPortType=input  RightPortType=output  PseudoPeriodic=off  Frequencies=[]  Unit=N*m  AffineConversion=off
  PS-Simulink Converter5 : nesl_utility/PS-Simulink Converter  PhysicalDomain=network_engine_domain  SubClassName=ps_output  LeftPortType=input  RightPortType=output  PseudoPeriodic=off  Frequencies=[]  Unit=rad  AffineConversion=off
  PS-Simulink Converter6 : nesl_utility/PS-Simulink Converter  PhysicalDomain=network_engine_domain  SubClassName=ps_output  LeftPortType=input  RightPortType=output  PseudoPeriodic=off  Frequencies=[]  Unit=N*m  AffineConversion=off
  PS-Simulink Converter7 : nesl_utility/PS-Simulink Converter  PhysicalDomain=network_engine_domain  SubClassName=ps_output  LeftPortType=input  RightPortType=output  PseudoPeriodic=off  Frequencies=[]  Unit=rad/s  AffineConversion=off
  PS-Simulink Converter8 : nesl_utility/PS-Simulink Converter  PhysicalDomain=network_engine_domain  SubClassName=ps_output  LeftPortType=input  RightPortType=output  PseudoPeriodic=off  Frequencies=[]  Unit=N*m  AffineConversion=off
  ReferenceFrame : sm_lib/Frames and Transforms/Reference Frame  BlockFunction=simmechanics.library.frames_transforms.reference_frame
  Revolute Joint1 : sm_lib/Joints/Revolute Joint  SenseConstraintForce=off  SenseConstraintForceX=off  SenseConstraintForceY=off  SenseConstraintForceZ=off  SenseConstraintTorque=off  SenseConstraintTorqueX=off  SenseConstraintTorqueY=off  SenseConstraintTorqueZ=off  SenseTotalForce=off  SenseTotalForceX=off  SenseTotalForceY=off  SenseTotalForceZ=off  SenseTotalTorque=off  SenseTotalTorqueX=off  SenseTotalTorqueY=off  SenseTotalTorqueZ=off  CompositeWrenchDir=FollowerOnBase  CompositeWrenchFrame=BaseFrame  EquilibriumPosition=0  EquilibriumPositionUnits=deg  SpringStiffness=spring_stiff  SpringStiffnessUnits=N*m/deg  DampingCoefficient=damping_coeff  DampingCoefficientUnits=N*m/(deg/s)  TorqueActuationMode=InputTorque  MotionActuationMode=ComputedMotion  SensePosition=on  SenseVelocity=on  SenseAcceleration=off  SenseTorqueForce=on  PositionTargetValue=0  PositionTargetValueUnits=deg  PositionTargetSpecify=off  PositionTargetPriority=High  VelocityTargetValue=0  VelocityTargetValueUnits=deg/s  VelocityTargetSpecify=off  VelocityTargetPriority=High  BlockFunction=simmechanics.library.joints.revolute_joint
  Revolute Joint2 : sm_lib/Joints/Revolute Joint  SenseConstraintForce=off  SenseConstraintForceX=off  SenseConstraintForceY=off  SenseConstraintForceZ=off  SenseConstraintTorque=off  SenseConstraintTorqueX=off  SenseConstraintTorqueY=off  SenseConstraintTorqueZ=off  SenseTotalForce=off  SenseTotalForceX=off  SenseTotalForceY=off  SenseTotalForceZ=off  SenseTotalTorque=off  SenseTotalTorqueX=off  SenseTotalTorqueY=off  SenseTotalTorqueZ=off  CompositeWrenchDir=FollowerOnBase  CompositeWrenchFrame=BaseFrame  EquilibriumPosition=0  EquilibriumPositionUnits=deg  SpringStiffness=spring_stiff  SpringStiffnessUnits=N*m/deg  DampingCoefficient=damping_coeff  DampingCoefficientUnits=N*m/(deg/s)  TorqueActuationMode=InputTorque  MotionActuationMode=ComputedMotion  SensePosition=on  SenseVelocity=on  SenseAcceleration=off  SenseTorqueForce=on  PositionTargetValue=0  PositionTargetValueUnits=deg  PositionTargetSpecify=off  PositionTargetPriority=High  VelocityTargetValue=0  VelocityTargetValueUnits=deg/s  VelocityTargetSpecify=off  VelocityTargetPriority=High  BlockFunction=simmechanics.library.joints.revolute_joint
  Revolute Joint3 : sm_lib/Joints/Revolute Joint  SenseConstraintForce=off  SenseConstraintForceX=off  SenseConstraintForceY=off  SenseConstraintForceZ=off  SenseConstraintTorque=off  SenseConstraintTorqueX=off  SenseConstraintTorqueY=off  SenseConstraintTorqueZ=off  SenseTotalForce=off  SenseTotalForceX=off  SenseTotalForceY=off  SenseTotalForceZ=off  SenseTotalTorque=off  SenseTotalTorqueX=off  SenseTotalTorqueY=off  SenseTotalTorqueZ=off  CompositeWrenchDir=FollowerOnBase  CompositeWrenchFrame=BaseFrame  EquilibriumPosition=0  EquilibriumPositionUnits=deg  SpringStiffness=spring_stiff  SpringStiffnessUnits=N*m/deg  DampingCoefficient=damping_coeff  DampingCoefficientUnits=N*m/(deg/s)  TorqueActuationMode=InputTorque  MotionActuationMode=ComputedMotion  SensePosition=on  SenseVelocity=on  SenseAcceleration=off  SenseTorqueForce=on  PositionTargetValue=0  PositionTargetValueUnits=deg  PositionTargetSpecify=off  PositionTargetPriority=High  VelocityTargetValue=0  VelocityTargetValueUnits=deg/s  VelocityTargetSpecify=off  VelocityTargetPriority=High  BlockFunction=simmechanics.library.joints.revolute_joint
  Tibia_left_3_RIGID : Subsystem
  F : PMIOPort  Port=1  Side=Right
  A1 : PMIOPort  Port=2  Side=Left
  A2 : PMIOPort  Port=3  Side=Left
  A3 : PMIOPort  Port=4  Side=Left
  F_GC : PMIOPort  Port=5  Side=Left
  S1 : Outport
  S2 : Outport  Port=2
  S3 : Outport  Port=3
  wires:
  Bus Creator/1 -> S3/1  "Servo3"
  PS-Simulink Converter1/1 -> Bus Creator/2  "Vel"
  PS-Simulink Converter/1 -> Bus Creator/1  "Pos"
  PS-Simulink Converter6/1 -> Bus Creator/3  "Torque"
  Bus Creator1/1 -> S2/1  "Servo2"
  PS-Simulink Converter3/1 -> Bus Creator1/2  "Vel"
  PS-Simulink Converter2/1 -> Bus Creator1/1  "Pos"
  PS-Simulink Converter4/1 -> Bus Creator1/3  "Torque"
  Bus Creator2/1 -> S1/1  "Servo1"
  PS-Simulink Converter7/1 -> Bus Creator2/2  "Vel"
  PS-Simulink Converter5/1 -> Bus Creator2/1  "Pos"
  PS-Simulink Converter8/1 -> Bus Creator2/3  "Torque"
  connections:
  A1/RConn1 -- Revolute Joint1/LConn2
  Coxa_left_3_RIGID1/LConn1 -- Revolute Joint1/RConn1
  ReferenceFrame/RConn1 -- Revolute Joint1/LConn1 -- F/RConn1
  F_GC/RConn1 -- Tibia_left_3_RIGID/RConn1
  Revolute Joint2/RConn1 -- Coxa_left_3_RIGID1/RConn1
  Revolute Joint3/LConn1 -- Tibia_left_3_RIGID/LConn1
  Revolute Joint3/RConn1 -- Femur_left_3_RIGID1/RConn1
  A2/RConn1 -- Revolute Joint2/LConn2
  PS-Simulink Converter2/LConn1 -- Revolute Joint2/RConn2
  PS-Simulink Converter3/LConn1 -- Revolute Joint2/RConn3
  PS-Simulink Converter4/LConn1 -- Revolute Joint2/RConn4
  A3/RConn1 -- Revolute Joint3/LConn2
  PS-Simulink Converter/LConn1 -- Revolute Joint3/RConn2
  PS-Simulink Converter1/LConn1 -- Revolute Joint3/RConn3
  PS-Simulink Converter6/LConn1 -- Revolute Joint3/RConn4
  Revolute Joint2/LConn1 -- Femur_left_3_RIGID1/LConn1
  PS-Simulink Converter8/LConn1 -- Revolute Joint1/RConn4
  PS-Simulink Converter7/LConn1 -- Revolute Joint1/RConn3
  PS-Simulink Converter5/LConn1 -- Revolute Joint1/RConn2
